simulink model "LIN_MORUS_GA"  (R2019a)
settings: Solver=ode45  StartTime=0.0  StopTime=t_sim  FixedStep=0.04  MaxStep=0.012  MinStep=1e-5  RelTol=1e-5  AbsTol=1e-10
values from neighbouring files (symbols this model uses):
  A_dis_calc = expm(kSamplingTime*A_continous_time)    [MPC_designer_X.m]    (also in NonTilting.m; RUN_simulation.m; Simulacija_MPC_YAW_NELINEARNI.m; Simulacija_MPC_Z.m)
  B_dis_calc = integral_exp_A * B_continous_time    [MPC_designer_X.m]    (also in NonTilting.m; RUN_simulation.m; Simulacija_MPC_YAW_NELINEARNI.m; Simulacija_MPC_Z.m)
  kSamplingTime = 0.810    (= 0.81)    [MPCDesigner_YAW.m]    (also in MPC_designer_X.m = 0.1; MPC_designer_Z.m; NonTilting.m = 0.015; RUN_simulation.m = 0.015)
  Q = inv(diag([0.5800 4*kSamplingTime 0.5800 4*kSamplingTime 300 300 0.2 (0.2/3) 100 4])) * diag([0, 0, 0, 0, 0, 0, 1e5,0, 1e7, 0]) *inv(diag([0.5800 4*kSamplingTime 0.5800 4*kSamplingTime 300 300 0.2 (0.2/3.0) 100 4]))    [NonTilting.m]    (also in RUN_simulation.m = diag([ 0.135340000000000,0.002706800000000,  0.1353400, 0.00; Simulacija_MPC_YAW_NELINEARNI.m = diag([pop(5),pop(6),pop(5),pop(6), pop(7),pop(7),pop(8),pop(; Simulacija_MPC_Z.m = diag([pop(5),pop(6),pop(5),pop(6), pop(7),pop(7),pop(8),pop(; Simulacija_Roll.m = diag([pop(5),pop(6),pop(5),pop(6), pop(7),pop(7),pop(8),pop()
  R = inv(diag([0.5800 0.5800 300 300]))*diag([0, 0, 0, 0])*inv(diag([0.5800 0.5800 300 300]))    [NonTilting.m]    (also in RUN_simulation.m = diag([0.67670, 0.67670, 0.13534000, 0.13534000]); Simulacija_MPC_YAW_NELINEARNI.m = diag([pop(1),pop(1),pop(2),pop(2)]); Simulacija_MPC_Z.m = diag([pop(1),pop(1),pop(2),pop(2)]); Simulacija_Roll.m = diag([pop(1),pop(1),pop(2),pop(2)]))
  R_delta = inv(diag([0.5800 0.5800 300 300]))* diag([0,0,0,0])*inv(diag([0.5800 0.5800 300 300]))    [NonTilting.m]    (also in RUN_simulation.m = diag([0.738879858135067, 0.738879858135067, 0.00738879858135; Simulacija_MPC_YAW_NELINEARNI.m = diag([pop(3),pop(3),pop(4),pop(4)]); Simulacija_MPC_Z.m = diag([pop(3),pop(3),pop(4),pop(4)]); Simulacija_Roll.m = diag([pop(3),pop(3),pop(4),pop(4)]))
  theta_x = pomocni    [Preuredi.m]
libraries: simulink x2
settings Model: Creator=branko  LastModifiedBy=branko
settings SolverCC: ConcurrentTasks=on
settings DataIOCC: ReturnWorkspaceOutputs=off
settings DebuggingCC: UnderSpecifiedDimensionMsg=warning  ArithmeticOperatorsInVariantConditions=warning

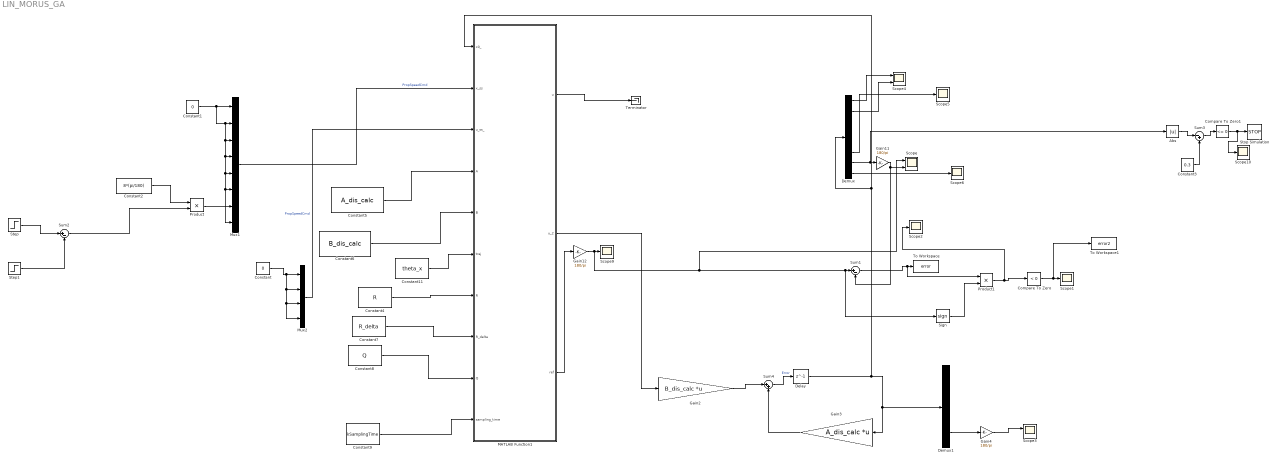
== system LIN_MORUS_GA ==
  Abs : Abs
  Compare To Zero : simulink/Logic and Bit Operations/Compare To Zero  relop=<  OutDataTypeStr=boolean
  Compare To Zero1 : simulink/Logic and Bit Operations/Compare To Zero  relop=<=  OutDataTypeStr=boolean
  Constant : Constant  Value=0  OutDataTypeStr=double  SampleTime=-1
  Constant1 : Constant  Value=0  OutDataTypeStr=double  SampleTime=-1
  Constant11 : Constant  Value=theta_x
  Constant2 : Constant  Value=8*(pi/180)  OutDataTypeStr=double
  Constant3 : Constant  Value=0.3  OutDataTypeStr=double
  Constant4 : Constant  Value=R
  Constant5 : Constant  Value=A_dis_calc
  Constant6 : Constant  Value=B_dis_calc
  Constant7 : Constant  Value=R_delta
  Constant8 : Constant  Value=Q
  Constant9 : Constant  Value=kSamplingTime
  Delay : Delay  DelayLength=1  SampleTime=kSamplingTime
  Demux : Demux  Outputs=8
  Demux1 : Demux  Outputs=8
  Gain11 : Gain  Gain=180/pi
  Gain12 : Gain  Gain=180/pi
  Gain2 : Gain  Gain=B_dis_calc  Multiplication=Matrix(K*u)
  Gain3 : Gain  Gain=A_dis_calc  Multiplication=Matrix(K*u)
  Gain4 : Gain  Gain=180/pi
  MATLAB Function1 : MATLAB Function  TreatAsAtomicUnit=on  SystemSampleTime=kSamplingTime
  Mux1 : Mux  Inputs=8
  Mux2 : Mux
  Product : Product
  Product1 : Product
  Scope : Scope  NumInputPorts=2
  Scope{1..2,5..6,9..10} (6 alike) : Scope
  Scope3 : Scope  NumInputPorts=2
  Scope4 : Scope  NumInputPorts=2
  Sign : Signum
  Step : Step  Time=0  SampleTime=0
  Step1 : Step  Time=15  After=2  SampleTime=0
  Stop Simulation : Stop
  Sum1 : Sum  Inputs=|+-
  Sum2 : Sum  Inputs=|+-
  Sum3 : Sum  Inputs=|-+
  Sum4 : Sum  Inputs=|++
  Terminator : Terminator
  To Workspace : ToWorkspace  VariableName=error  SaveFormat=Structure With Time  SampleTime=-1
  To Workspace1 : ToWorkspace  VariableName=error2  SaveFormat=Structure With Time  SampleTime=-1
  wires:
  Mux1/1 -> MATLAB Function1/2(x_ss)  "PropSpeedCmd"
  Mux2/1 -> MATLAB Function1/3(u_ss_)  "PropSpeedCmd"
  Constant/1 -> Mux2/4, Mux2/3, Mux2/2, Mux2/1
  Constant1/1 -> Mux1/6, Mux1/8, Mux1/5, Mux1/4, Mux1/3, Mux1/2, Mux1/1
  Demux/7 -> Abs/1, Gain11/1
  Step/1 -> Sum2/1
  Constant2/1 -> Product/1
  Sum2/1 -> Product/2
  Step1/1 -> Sum2/2
  Product/1 -> Mux1/7
  Constant5/1 -> MATLAB Function1/4(A)
  Constant6/1 -> MATLAB Function1/5(B)
  MATLAB Function1/2(u_2) -> Gain2/1
  Constant11/1 -> MATLAB Function1/6(traj)
  MATLAB Function1/3(ref) -> Gain12/1
  Gain12/1 -> Scope/1, Sign/1, Sum1/1, Scope9/1
  Sum1/1 -> Product1/1, To Workspace/1
  Sign/1 -> Product1/2
  Product1/1 -> Scope2/1, Compare To Zero/1
  Compare To Zero/1 -> To Workspace1/1, Scope1/1
  Compare To Zero1/1 -> Scope10/1, Stop Simulation/1
  Abs/1 -> Sum3/1
  Constant3/1 -> Sum3/2
  Gain11/1 -> Sum1/2, Scope/2
  Sum3/1 -> Compare To Zero1/1
  MATLAB Function1/1(u) -> Terminator/1
  Constant4/1 -> MATLAB Function1/7(R)
  Constant7/1 -> MATLAB Function1/8(R_delta)
  Constant8/1 -> MATLAB Function1/9(Q)
  Constant9/1 -> MATLAB Function1/10(sampling_time)
  Gain2/1 -> Sum4/1
  Gain3/1 -> Sum4/2
  Sum4/1 -> Delay/1  "Error"
  Delay/1 -> MATLAB Function1/1(x0_), Demux/1, Demux1/1, Gain3/1
  Demux1/7 -> Gain4/1
  Gain4/1 -> Scope3/1
  Demux/1 -> Scope4/1
  Demux/2 -> Scope4/2
  Demux/6 -> Scope5/1
  Demux/8 -> Scope6/1

== matlab function LIN_MORUS_GA/MATLAB Function1 ==
  settings: updateMethod=DISCRETE
  data: x0_ input; u output; x_ss input; u_ss_ input; u_2 output; A input; B input; traj input; ref output; R input; R_delta input; Q input; sampling_time input
function [u, u_2, ref]  = adam(x0_, x_ss, u_ss_, A, B, traj, R, R_delta, Q, sampling_time)

persistent new_desire_state  pred_horizon control_horizon max_iter  ...
           scale_MV_inv   scale_OV_inv gradients gradient_past ...
           gradient_square_past gradient_past_tilda gradient_square_past_tilda ...
           x_states deriv_wrt_u epsilon rho1 rho2 delta num_heuristic_vars ...
           u_past u_current lambdas_x lambdas_u lambdas_u_ref u_horizon ref_old t u_last_step ...
           du_max u_max index_first 



x_ss_ = 0* x_ss;


  
if(isempty(new_desire_state) )
%     counter = 3;
    index_first = 0;
    u_last_step = zeros(4, 1);
    du_max = zeros(4,2);
    u_max = zeros(4,2);
    
    du_max(1,1) = sampling_time* 2;
    du_max(1,2) = -sampling_time * 2;
    du_max(2,1) = sampling_time * 2;
    du_max(2,2) = -sampling_time * 2;
    du_max(3,1) = 1*(sampling_time/0.01);
    du_max(3,2) = -1*(sampling_time/0.01);
    du_max(4,1) = 1*(sampling_time/0.01);
    du_max(4,2) = -1*(sampling_time/0.01);
    
    u_max(1,1) = 0.6 / 2 - 0.01;
    u_max(1,2) = -u_max(1,1);
    u_max(2,1) = 0.6 / 2 - 0.01;
    u_max(2,2) = -u_max(1,1);
    u_max(3,1) = 50;
    u_max(3,2) = -50;
    u_max(4,1) = 50;
    u_max(4,2) = -50;
    
    ref_old  = x_ss_;
    t = 0.0;
    epsilon = 0.04;
	rho1 = 0.9;
	rho2 = 0.999;
	delta = 1e-7;
max_iter = 5;
control_horizon = 5;
pred_horizon = 14;
num_heuristic_vars = 2;
gradients = zeros(num_heuristic_vars*control_horizon,1 );
gradient_past = zeros(num_heuristic_vars*control_horizon,1 );
gradient_past_tilda = zeros(num_heuristic_vars*control_horizon,1 );
gradient_square_past_tilda = zeros(num_heuristic_vars*control_horizon,1 );
gradient_square_past = zeros(num_heuristic_vars*control_horizon,1 );
new_desire_state = true;
scale_OV_inv = inv(diag([0.58, 4.0, 0.58, 4.0, 800, 800, 0.5236, 0.5236]));

scale_MV_inv = inv(diag([0.58, 0.58, 100, 100]));

%old
% R =diag([0.67670, 0.67670, 0.13534000, 0.13534000]);
% R_delta = diag([0.738879858135067, 0.738879858135067, 0.007388798581351,0.007388798581351]);
% Q = diag([ 0.135340000000000,0.002706800000000,  0.1353400, 0.002706800, 0.002706800, 0.002706800,80.7068000, 9.676700]);



% 
% A =[    0.4271,    0.0223,         0,         0,         0,         0,         0 ,        0;
%    -8.7243,   -0.1501,         0,         0,         0,         0,         0,         0;
%          0,         0,    0.4271,    0.0223,         0,         0,         0,         0;
%          0,         0,   -8.7243,   -0.1501,         0,         0,         0,         0;
%          0,         0,         0,         0,    0.7300,         0,         0,         0;
%          0,         0,         0,         0,         0,    0.7300,         0,         0;
%     0.0090,    0.0005,    0.0090,    0.0005,    0.0001,   -0.0001,    1.0000,    0.0787;
%     0.1699,    0.0113,    0.1699,    0.0113,    0.0028,   -0.0028,         0 ,   1.0000];
%     
% B =[ 0.5729,         0 ,        0 ,        0;
%     8.7243,         0   ,      0 ,        0;
%          0,    0.5729  ,       0 ,        0;
%          0,    8.7243 ,        0 ,        0;
%          0,         0 ,   0.2700 ,        0;
%          0,         0 ,        0 ,   0.2700;
%    -0.0037,   -0.0037,    0.0000 ,  -0.0000;
%    -0.0347,   -0.0347,    0.0005 ,  -0.0005];



x_states = zeros(size(A, 1), pred_horizon+1);
deriv_wrt_u =  zeros(size(B,2), control_horizon);
u_past = zeros(size(B,2), 1);
u_current = zeros(size(B,2), 1);
u_ss_ = zeros(size(B,2), 1);
lambdas_x = zeros(size(A, 1), pred_horizon);
lambdas_u = zeros(size(B,2), pred_horizon);
u_horizon = zeros(size(B,2), pred_horizon);
lambdas_u_ref = zeros(size(B,2), pred_horizon);

end
if(index_first == 70)
index_first
end

size(x0_)

if(index_first < length(traj))
    if(abs(x0_(7) - traj(index_first +1)) < 0.12 )
        index_first = index_first +1;
        new_desire_state = true;
    end
end



        
if(index_first < length(traj))
    ref = traj(1 + index_first);
else
    ref  = 0.0;
end
residuum_signal =0.0;
residuum_state =0.0;

u = zeros(size(B,2), 1);

x = zeros(control_horizon *num_heuristic_vars,1);
change_x = zeros(control_horizon *num_heuristic_vars,1);

% if(sum(x_ss_ - ref_old, 'double') < 1e-6)
%    new_desire_state = false; 
% else
%     new_desire_state = true;
% 
% end

% if(mod(index_first,3)== 0)
%      new_desire_state = true;
% end
new_desire_state = true;
for iter = 1:max_iter
x_states(:,1) = x0_ ;
deriv_wrt_u = 0*deriv_wrt_u;
u_past = zeros(size(B,2), 1);% u_current*1;

if (new_desire_state) 
		new_desire_state = false;
		gradient_past = 0*gradient_past;
		gradient_square_past = 0*gradient_square_past;
		t = 0.0;
end

for i = 1:pred_horizon
    
    if(i <= control_horizon)
        u(1,1) = x(0*control_horizon  + i);
        u(2,1) = x(0*control_horizon  + i);
        u(3,1) = x(1*control_horizon  + i);
        u(4,1) = -x(1*control_horizon  + i);
    end
    
    if((index_first + i) > length(traj))
            x_ss_(7) = 0.0;
            x_ss_(8) = 0.0;
    else
            x_ss_(7) = traj(index_first+i);
%             if(index_first > 1)
%              x_ss_(8) = ( traj(index_first + i) - traj(index_first + i-1) )/0.01;
%             else
%                  x_ss_(8) = ( traj(index_first + i)  )/0.01;
%             end
    end
    
    x_states(:,i+1) = A * x_states(:,i) + B * u; 
    lambdas_x(:,i) = -1*x_ss_ + x_states(:,i+1); 
    lambdas_u(:,i) = u - u_past; 
    lambdas_u_ref(:, i) = u - u_ss_; 
 
    %derivation of u
    if(i <= control_horizon)
        deriv_wrt_u(:, i) = (2*R*u) -2*R*u_ss_  + (4*R_delta*u) -2*R_delta*u_past + deriv_wrt_u(:, i) ;
        
        if(i > 1)
            deriv_wrt_u(:, i-1) = deriv_wrt_u(:, i-1) -2*R_delta*u ;
        end
    else
        deriv_wrt_u(:, control_horizon) = deriv_wrt_u(:, control_horizon) + (2*R*u) -2*R*u_ss_  + (4*R_delta*u)+ (-2*R_delta*u_past) ;
        deriv_wrt_u(:, control_horizon) = deriv_wrt_u(:, control_horizon) -2*R_delta*u ;
    end
    
    %derivation of x
    for j = 1:i
        if(j <= control_horizon && i <= control_horizon)
            
            deriv_wrt_u(:,j) = deriv_wrt_u(:,j) + transpose(transpose( 2*Q*x_states(:,i+1) - 2*Q*x_ss_ )*(A^(i-j))*B); 
        else
            if(j > control_horizon)
                deriv_wrt_u(:,control_horizon) =deriv_wrt_u(:,control_horizon) +  transpose(transpose((2*Q*x_states(:,i+1) - 2*Q*x_ss_))*(A^(i-j))*B); 
            else
                deriv_wrt_u(:,j) =deriv_wrt_u(:,j) + transpose(transpose( 2*Q*x_states(:,i+1) - 2*Q*x_ss_ )*(A^(i-j))*B); 
            end
        end
    end
    u_past = u;
end


lambdas_u_ref =scale_MV_inv * lambdas_u_ref;
lambdas_u = scale_MV_inv * lambdas_u;
lambdas_x = scale_OV_inv * lambdas_x;
residuum_signal=sum((lambdas_u_ref.*(R*lambdas_u_ref)),'double')  + sum((lambdas_u.*(R_delta*lambdas_u)),'double'); 
residuum_state=sum((lambdas_x.*(Q*lambdas_x)),'double') ; 
        
residuum =  residuum_signal +  residuum_state;

for iter_der = 1:control_horizon
    gradients(iter_der, 1) = 2 * deriv_wrt_u(1, iter_der);
    gradients(iter_der + control_horizon, 1) = 2 * deriv_wrt_u(3, iter_der);
end

gradient_square_past = (rho2*gradient_square_past + (1 - rho2)*gradients.*(gradients));

gradient_past = (rho1*gradient_past + (1 - rho1)*gradients);

t  = t +1.0;

for adam_iter = 1:control_horizon *num_heuristic_vars
    gradient_past_tilda(adam_iter, 1) = (gradient_past(adam_iter, 1)) / (1.0 - (rho1^t));
	gradient_square_past_tilda(adam_iter, 1) = (gradient_square_past(adam_iter, 1)) / (1.0 - (rho2^t));
		

end

for adam_iter = 1:control_horizon *num_heuristic_vars
    change_x(adam_iter, 1) = -1 * (epsilon * gradient_past_tilda(adam_iter, 1)) / (sqrt(gradient_square_past_tilda(adam_iter, 1)) + delta);

end

x = (x + change_x);
end

u(1,1) = x(0*control_horizon  + 1);
u(2,1) = x(0*control_horizon  + 1);
u(3,1) = x(1*control_horizon  + 1);
u(4,1) = -x(1*control_horizon  + 1);
x(1:control_horizon-1) = x(2:control_horizon);
x(control_horizon:2*control_horizon -1) = x(control_horizon +1:2*control_horizon)
u_2 = u;
for iter_m = 1:4
    if(u_2(iter_m,1) > ( u_last_step(iter_m,1)+du_max(iter_m,1) ))
        u_2(iter_m,1) =  u_last_step(iter_m,1)+du_max(iter_m,1);
    elseif (u_2(iter_m,1) < ( u_last_step(iter_m,1)+du_max(iter_m,2) ))
        u_2(iter_m,1) =  u_last_step(iter_m,1)+du_max(iter_m,2);
    end
    
    if(u_2(iter_m,1) > u_max(iter_m,1) )
        u_2(iter_m,1) =  u_max(iter_m,1);
    elseif(u_2(iter_m,1) < u_max(iter_m,2))
        u_2(iter_m,1) =  u_max(iter_m,2);
    end
    
    
end


u_last_step = u_2;
end
